simulink model "iopid_clamping"  (R2017a)
settings: Solver=FixedStepAuto  StartTime=0.0  StopTime=100  FixedStep=0.01  RelTol=1e-3
undefined symbols (not defined in the file): CoordinateFrame, TypeMask, Velocity
libraries: robotlib x3, simulink x1
settings Model: Creator=bshang2  LastModifiedBy=bshang2

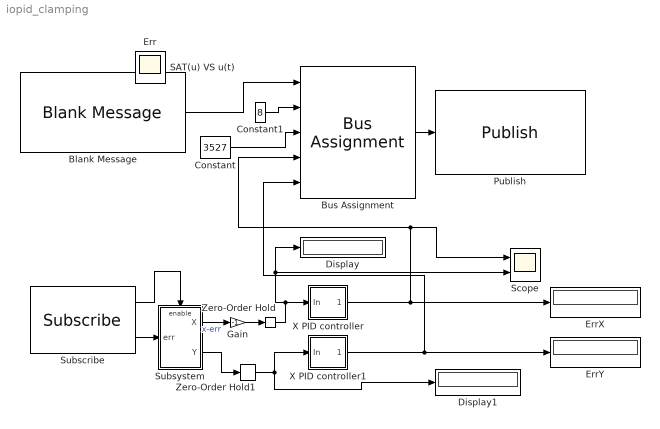
== system iopid_clamping ==
  Blank Message : robotlib/Blank Message  SourceLibraryInfo=This block requires Robotics System Toolbox  messageType=mavros_msgs/PositionTarget  SampleTime=inf
      settings: SourceProductBaseCode=RO
  Bus Assignment : BusAssignment  AssignedSignals=CoordinateFrame,TypeMask,Velocity.X,Velocity.Y
  Constant : Constant  Value=3527  OutDataTypeStr=uint16
  Constant1 : Constant  Value=8  OutDataTypeStr=uint8
  Display : Display
  Display1 : Display
  ErrX : Display
  ErrY : Display
  Gain : Gain  Gain=-1
  Publish : robotlib/Publish  SourceLibraryInfo=This block requires Robotics System Toolbox  topicSource=Select from ROS network  topic=/mavros/setpoint_raw/local  messageType=mavros_msgs/PositionTarget  messageQueueLength=1
      settings: SourceProductBaseCode=RO
  Scope : Scope  NumInputPorts=2
  Subscribe : robotlib/Subscribe  SourceLibraryInfo=This block requires Robotics System Toolbox  topicSource=Select from ROS network  topic=/matlab/err  messageType=geometry_msgs/Pose2D  sampleTime=-1  messageQueueLength=1
      settings: SourceProductBaseCode=RO
  Subsystem : Subsystem
  X PID controller : Subsystem
  X PID controller1 : Subsystem
  Zero-Order Hold : ZeroOrderHold  SampleTime=-1
  Zero-Order Hold1 : ZeroOrderHold  SampleTime=-1
  Err : Scope
  SAT(u) VS u(t) : Scope
  wires:
  Blank Message/1 -> Bus Assignment/1
  X PID controller/1(Out) -> ErrX/1, Scope/1, Bus Assignment/4
  Bus Assignment/1 -> Publish/1
  Subscribe/2 -> Subsystem/1(err)
  Subsystem/1(X) -> Gain/1  "x-err"
  Subsystem/2(Y) -> Zero-Order Hold1/1
  Subscribe/1 -> Subsystem/Enable
  X PID controller1/1(Out) -> Bus Assignment/5, ErrY/1
  Constant/1 -> Bus Assignment/3
  Constant1/1 -> Bus Assignment/2
  Zero-Order Hold/1 -> Display/1, Scope/2, X PID controller/1(In)
  Zero-Order Hold1/1 -> X PID controller1/1(In), Display1/1
  Gain/1 -> Zero-Order Hold/1

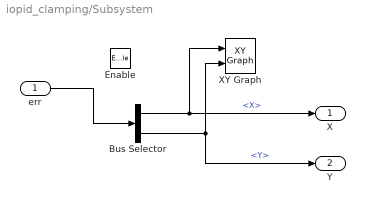
== system iopid_clamping/Subsystem ==
  err : Inport
  Enable : EnablePort
  Bus Selector : BusSelector  OutputSignals=X,Y
  XY Graph : simulink/Sinks/XY Graph  xmin=-100  xmax=100  ymin=-100  ymax=100  st=-1
  X : Outport
  Y : Outport  Port=2
  wires:
  err/1 -> Bus Selector/1
  Bus Selector/1 -> X/1, XY Graph/1  "<X>"
  Bus Selector/2 -> Y/1, XY Graph/2  "<Y>"

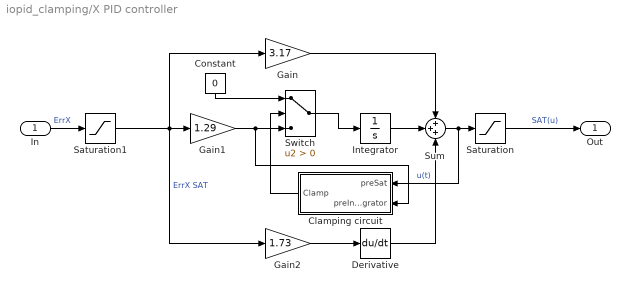
== system iopid_clamping/X PID controller ==
  In : Inport
  Clamping circuit : Subsystem
  Constant : Constant  DisableCoverage=on  Value=0  OutDataTypeStr=Inherit: Inherit via back propagation  PreserveConstantTs=on
  Derivative : Derivative
  Gain : Gain  Gain=3.17
  Gain1 : Gain  Gain=1.29
  Gain2 : Gain  Gain=1.73
  Integrator : Integrator
  Saturation : Saturate  UpperLimit=0.3  LowerLimit=-0.3
  Saturation1 : Saturate  UpperLimit=200  LowerLimit=-200
  Sum : Sum  Inputs=+++
  Switch : Switch  Criteria=u2 > Threshold  SaturateOnIntegerOverflow=on  InputSameDT=on
  Out : Outport
  wires:
  Sum/1 -> Clamping circuit/1(preSat), Saturation/1  "u(t)"
  In/1 -> Saturation1/1  "ErrX"
  Gain1/1 -> Clamping circuit/2(preIntegrator), Switch/3
  Gain2/1 -> Derivative/1
  Gain/1 -> Sum/1
  Integrator/1 -> Sum/2
  Derivative/1 -> Sum/3
  Saturation/1 -> Out/1  "SAT(u)"
  Switch/1 -> Integrator/1
  Saturation1/1 -> Gain1/1, Gain2/1, Gain/1  "ErrX SAT"
  Clamping circuit/1(Clamp) -> Switch/2
  Constant/1 -> Switch/1

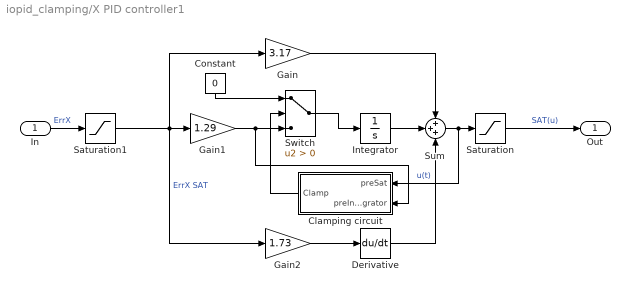
== system iopid_clamping/X PID controller1 ==
  In : Inport
  Clamping circuit : Subsystem
  Constant : Constant  DisableCoverage=on  Value=0  OutDataTypeStr=Inherit: Inherit via back propagation  PreserveConstantTs=on
  Derivative : Derivative
  Gain : Gain  Gain=3.17
  Gain1 : Gain  Gain=1.29
  Gain2 : Gain  Gain=1.73
  Integrator : Integrator
  Saturation : Saturate  UpperLimit=0.3  LowerLimit=-0.3
  Saturation1 : Saturate  UpperLimit=0.3  LowerLimit=-0.3
  Sum : Sum  Inputs=+++
  Switch : Switch  Criteria=u2 > Threshold  SaturateOnIntegerOverflow=on  InputSameDT=on
  Out : Outport
  wires:
  Sum/1 -> Clamping circuit/1(preSat), Saturation/1  "u(t)"
  In/1 -> Saturation1/1  "ErrX"
  Gain1/1 -> Clamping circuit/2(preIntegrator), Switch/3
  Gain2/1 -> Derivative/1
  Gain/1 -> Sum/1
  Integrator/1 -> Sum/2
  Derivative/1 -> Sum/3
  Saturation/1 -> Out/1  "SAT(u)"
  Switch/1 -> Integrator/1
  Saturation1/1 -> Gain1/1, Gain2/1, Gain/1  "ErrX SAT"
  Clamping circuit/1(Clamp) -> Switch/2
  Constant/1 -> Switch/1

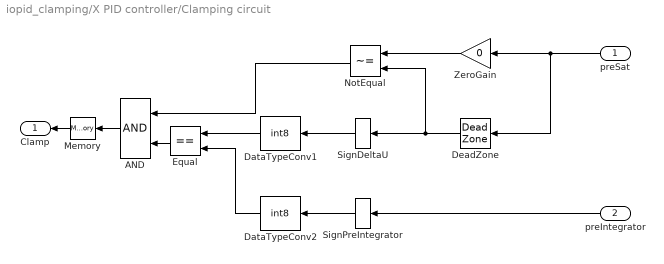
== system iopid_clamping/X PID controller/Clamping circuit ==
  preSat : Inport  DisableCoverage=on
  preIntegrator : Inport  DisableCoverage=on  Port=2
  AND : Logic  DisableCoverage=on
  DataTypeConv1 : DataTypeConversion  DisableCoverage=on  OutDataTypeStr=int8  SaturateOnIntegerOverflow=on  RndMeth=Zero  LockScale=on
  DataTypeConv2 : DataTypeConversion  DisableCoverage=on  OutDataTypeStr=int8  SaturateOnIntegerOverflow=on  RndMeth=Zero  LockScale=on
  DeadZone : DeadZone  DisableCoverage=on  LowerValue=-0.3  UpperValue=0.3  SaturateOnIntegerOverflow=on
  Equal : RelationalOperator  DisableCoverage=on  Operator===  RndMeth=Nearest  InputSameDT=on
  Memory : Memory  DisableCoverage=on
  NotEqual : RelationalOperator  DisableCoverage=on  Operator=~=  RndMeth=Nearest  InputSameDT=on
  SignDeltaU : Signum  DisableCoverage=on
  SignPreIntegrator : Signum  DisableCoverage=on
  ZeroGain : Gain  DisableCoverage=on  Gain=0  SaturateOnIntegerOverflow=on  OutDataTypeStr=Inherit: Same as input  ParamDataTypeStr=Inherit: Same as input
  Clamp : Outport  DisableCoverage=on
  wires:
  preSat/1 -> ZeroGain/1, DeadZone/1
  preIntegrator/1 -> SignPreIntegrator/1
  ZeroGain/1 -> NotEqual/1
  DeadZone/1 -> NotEqual/2, SignDeltaU/1
  SignDeltaU/1 -> DataTypeConv1/1
  DataTypeConv1/1 -> Equal/1
  SignPreIntegrator/1 -> DataTypeConv2/1
  DataTypeConv2/1 -> Equal/2
  NotEqual/1 -> AND/1
  Equal/1 -> AND/2
  AND/1 -> Memory/1
  Memory/1 -> Clamp/1

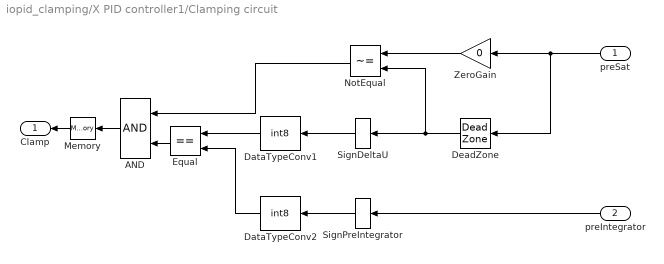
== system iopid_clamping/X PID controller1/Clamping circuit ==
  preSat : Inport  DisableCoverage=on
  preIntegrator : Inport  DisableCoverage=on  Port=2
  AND : Logic  DisableCoverage=on
  DataTypeConv1 : DataTypeConversion  DisableCoverage=on  OutDataTypeStr=int8  SaturateOnIntegerOverflow=on  RndMeth=Zero  LockScale=on
  DataTypeConv2 : DataTypeConversion  DisableCoverage=on  OutDataTypeStr=int8  SaturateOnIntegerOverflow=on  RndMeth=Zero  LockScale=on
  DeadZone : DeadZone  DisableCoverage=on  LowerValue=-0.3  UpperValue=0.3  SaturateOnIntegerOverflow=on
  Equal : RelationalOperator  DisableCoverage=on  Operator===  RndMeth=Nearest  InputSameDT=on
  Memory : Memory  DisableCoverage=on
  NotEqual : RelationalOperator  DisableCoverage=on  Operator=~=  RndMeth=Nearest  InputSameDT=on
  SignDeltaU : Signum  DisableCoverage=on
  SignPreIntegrator : Signum  DisableCoverage=on
  ZeroGain : Gain  DisableCoverage=on  Gain=0  SaturateOnIntegerOverflow=on  OutDataTypeStr=Inherit: Same as input  ParamDataTypeStr=Inherit: Same as input
  Clamp : Outport  DisableCoverage=on
  wires:
  preSat/1 -> ZeroGain/1, DeadZone/1
  preIntegrator/1 -> SignPreIntegrator/1
  ZeroGain/1 -> NotEqual/1
  DeadZone/1 -> NotEqual/2, SignDeltaU/1
  SignDeltaU/1 -> DataTypeConv1/1
  DataTypeConv1/1 -> Equal/1
  SignPreIntegrator/1 -> DataTypeConv2/1
  DataTypeConv2/1 -> Equal/2
  NotEqual/1 -> AND/1
  Equal/1 -> AND/2
  AND/1 -> Memory/1
  Memory/1 -> Clamp/1
